simulink model "simulink2"  (R2023a)
settings: Solver=VariableStepAuto  StartTime=0.0  StopTime=10.0  RelTol=1e-3
settings Model: Creator=94410  LastModifiedBy=94410

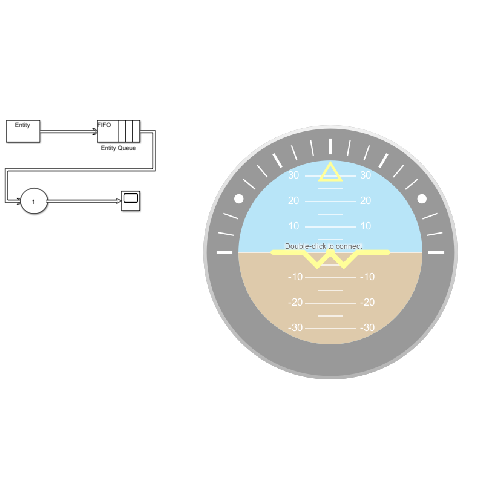
[thumbnail: Simulink's stored preview of the top-level diagram]
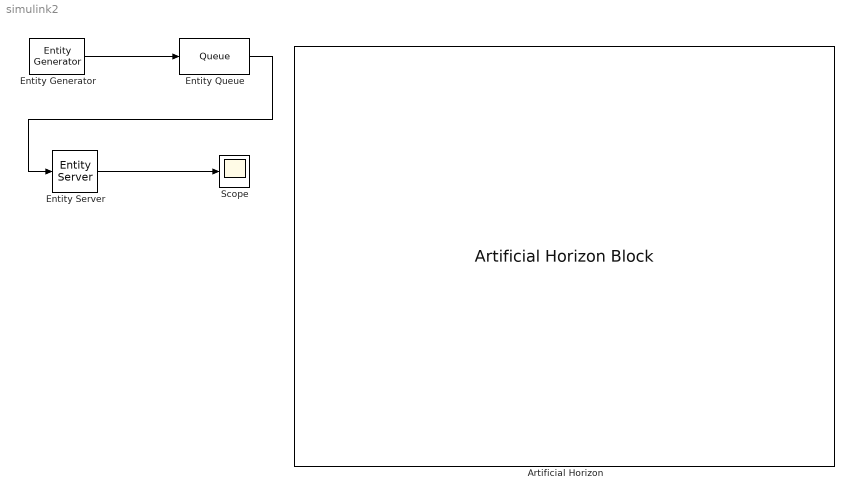
== system simulink2 ==
  Artificial Horizon : ArtificialHorizonBlock  LabelPosition=Hide
  Entity Generator : EntityGenerator  OutputPortMessageModes=m  EntityType=Structured  EntityTypeName=Entity
  Entity Queue : Queue  InputPortMessageModes=m  OutputPortMessageModes=m
  Entity Server : EntityServer  InputPortMessageModes=m  OutputPortMessageModes=m  Capacity=1
  Scope : Scope
  wires:
  Entity Generator/1 -> Entity Queue/1
  Entity Queue/1 -> Entity Server/1
  Entity Server/1 -> Scope/1
